simulink model "EthernetMicro"  (R2015b)
settings: Solver=FixedStepDiscrete  StartTime=0.0  StopTime=inf  RelTol=1e-3
libraries: xpcutilitieslib x1, arduinolib x1, arduinoethernetlib x1
settings Model: ExtModeTrigDuration=2  Creator=User  LastModifiedBy=User
settings OptimizationCC: OptimizeModelRefInitCode=on  LifeSpan=1  MaxStackSize=64
settings HardwareCC: ProdBitPerInt=16  ProdBitPerPointer=16  ProdLargestAtomicFloat=None  ProdWordSize=8  ProdHWDeviceType=Atmel->AVR
settings RTWCC: SystemTargetFile=ert.tlc  TemplateMakefile=ert_default_tmf  Description=Embedded Coder  Toolchain=Arduino AVR v1.6.1  BuildConfiguration=Faster Runs
settings CodeAppCC: IgnoreCustomStorageClasses=off
settings ERTTargetCC: SupportContinuousTime=on  SupportVariableSizeSignals=on

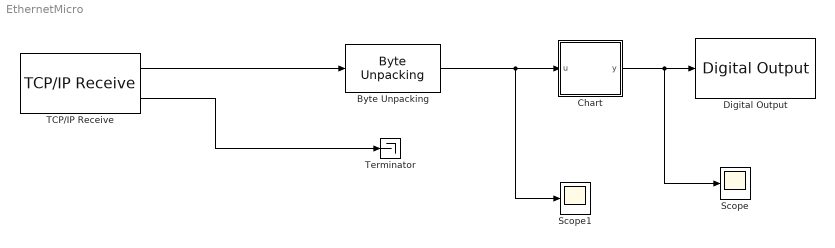
== system EthernetMicro ==
  "Byte Unpacking " : xpcutilitieslib/Byte Unpacking   MaskUnpackedDataTypes={'uint8'}  MaskUnpackedDataSizes={[1]}  MaskAlignment=1
  Chart : Stateflow chart  TreatAsAtomicUnit=on
  Digital Output : arduinolib/Digital Output  pinNumber=9  blockPlatform=arduino
  Scope : Scope
  Scope1 : Scope
  TCP/IP Receive : arduinoethernetlib/TCP//IP Receive  serverport=5896  sampleTime=1  blockPlatform=arduino
  Terminator : Terminator
  wires:
  "Byte Unpacking "/1 -> Scope1/1, Chart/1(u)
  Chart/1(y) -> Scope/1, Digital Output/1
  TCP/IP Receive/2 -> Terminator/1
  TCP/IP Receive/1 -> "Byte Unpacking "/1

== stateflow chart EthernetMicro/Chart ==
  state Off
    entry: y=0
  state On
    entry: y = 1
  (default) -> On
  On -> Off : [u<=5]
  Off -> On : [u>5]
  data: u input; y output
